simulink model "DC_MOTOR"  (R2019b)
settings: Solver=VariableStepAuto  StartTime=0.0  StopTime=1.0  RelTol=1e-3
undefined symbols (not defined in the file): Fm, G, Im, k_gear, kt, kv, La, Ml, Ra, Rl
settings Model: Creator=simone  LastModifiedBy=simone

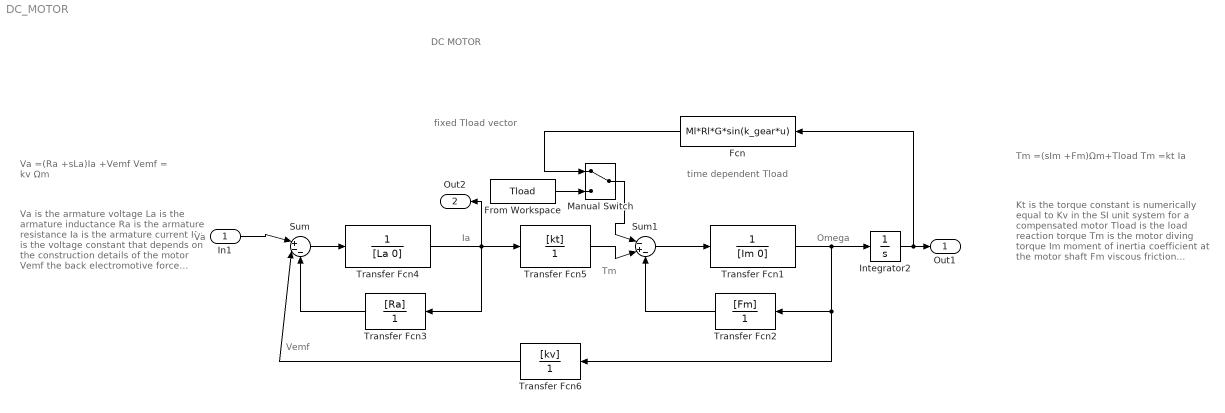
== system DC_MOTOR ==
  note: fixed Tload vector
  note: time dependent Tload
  note: DC MOTOR
  note: Va is the armature voltage
      |
      | La is the armature inductance
      |
      | Ra is the armature resistance
      |
      | Ia is the armature current
      |
      | Kv is the voltage constant that
      | depends on the construction
      | details of the motor
      |
      | Vemf the back electromotive force
      | which is proportional to the
      | angular velocity Ωm through the
      | voltage constant Kv
      |
      | 1/s is laplace domain integer
  note: Tm =(sIm +Fm)Ωm+Tload
      |
      | Tm =kt Ia
  note: Kt is the torque constant is numerically
      | equal to Kv in the SI unit system for a
      | compensated motor
      |
      | Tload is the load reaction torque
      |
      | Tm is the motor diving torque
      |
      | Im moment of inertia coefficient at the
      | motor shaft
      |
      | Fm viscous friction coefficient at the
      | motor shaft
      |
      | Omega is the angular velocity
      |
      | Theta is the angular position
  note: Va
  note: Tm
  note: Vemf
  note: Omega
  note: Ia
  note: Va =(Ra +sLa)Ia +Vemf
      |
      | Vemf = kv Ωm
  In1 : Inport
  Fcn : Fcn  Expr=Ml*Rl*G*sin(k_gear*u)
  From Workspace : FromWorkspace  VariableName=Tload  SampleTime=0.01
  Integrator2 : Integrator
  Manual Switch : ManualSwitch
  Sum : Sum  Inputs=|+--
  Sum1 : Sum  Inputs=|-+-
  Transfer Fcn1 : TransferFcn  Denominator=[Im 0]  ContinuousStateAttributes="\"\""
  Transfer Fcn2 : TransferFcn  Numerator=[Fm]  Denominator=[1]  ContinuousStateAttributes="\""
  Transfer Fcn3 : TransferFcn  Numerator=[Ra]  Denominator=[1]  ContinuousStateAttributes="\""
  Transfer Fcn4 : TransferFcn  Denominator=[La 0]  ContinuousStateAttributes="\"\""
  Transfer Fcn5 : TransferFcn  Numerator=[kt]  Denominator=[1]  ContinuousStateAttributes="\""
  Transfer Fcn6 : TransferFcn  Numerator=[kv]  Denominator=[1]  ContinuousStateAttributes="\""
  Out1 : Outport  SignalName=Theta
  Out2 : Outport  Port=2  SignalName=Ia
  wires:
  Sum/1 -> Transfer Fcn4/1
  Transfer Fcn4/1 -> Transfer Fcn5/1, Transfer Fcn3/1, Out2/1
  Transfer Fcn3/1 -> Sum/3
  Transfer Fcn2/1 -> Sum1/3
  Integrator2/1 -> Fcn/1, Out1/1
  Transfer Fcn6/1 -> Sum/2
  Sum1/1 -> Transfer Fcn1/1
  Transfer Fcn5/1 -> Sum1/2
  In1/1 -> Sum/1
  From Workspace/1 -> Manual Switch/2
  Fcn/1 -> Manual Switch/1
  Manual Switch/1 -> Sum1/1
  Transfer Fcn1/1 -> Integrator2/1, Transfer Fcn6/1, Transfer Fcn2/1
